simulink subsystem "KinematicModel"  (R2023b)
settings: Solver=VariableStepAuto  StartTime=0.0  StopTime=10.0  RelTol=1e-3
undefined symbols (not defined in the file): EOL_Vehicle_INITR, EOL_Vehicle_InitX, EOL_Vehicle_InitY, EOL_Vehicle_lf, EOL_Vehicle_lr
settings Model: Creator=konur  LastModifiedBy=konur

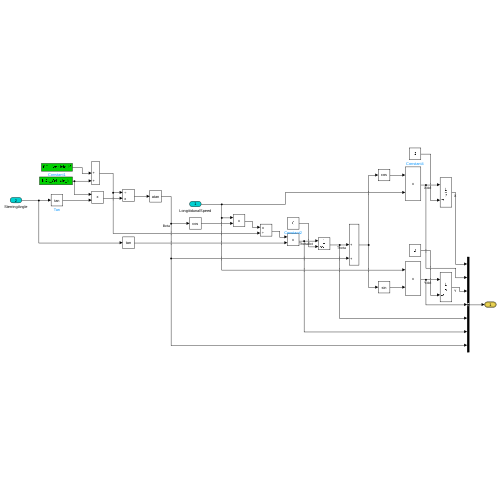
[thumbnail: Simulink's stored preview of the top-level diagram]
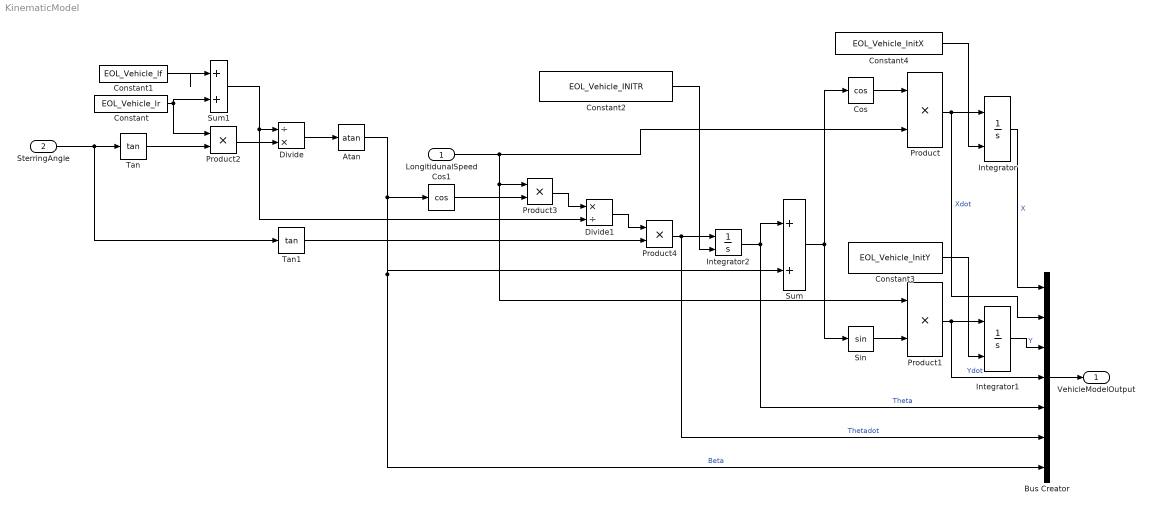
== system KinematicModel ==
  LongitidunalSpeed : Inport
  SterringAngle : Inport  Port=2
  Atan : Trigonometry  Operator=atan
  Bus Creator : BusCreator  Inputs=7  OutDataTypeStr=Bus: VehicleModelBus  NonVirtualBus=on
  Constant : Constant  Value=EOL_Vehicle_lr  OutDataTypeStr=double
  Constant1 : Constant  Value=EOL_Vehicle_lf  OutDataTypeStr=double
  Constant2 : Constant  Value=EOL_Vehicle_INITR  OutDataTypeStr=double
  Constant3 : Constant  Value=EOL_Vehicle_InitY  OutDataTypeStr=double
  Constant4 : Constant  Value=EOL_Vehicle_InitX  OutDataTypeStr=double
  Cos : Trigonometry  Operator=cos
  Cos1 : Trigonometry  Operator=cos
  Divide : Product  Inputs=/*  OutDataTypeStr=double
  Divide1 : Product  Inputs=*/
  Integrator : Integrator  InitialConditionSource=external
  Integrator1 : Integrator  InitialConditionSource=external
  Integrator2 : Integrator  InitialConditionSource=external
  Product{,1..4} (5 alike) : Product
  Sin : Trigonometry
  Sum : Sum  Inputs=|++  OutDataTypeStr=double
  Sum1 : Sum  Inputs=|++  OutDataTypeStr=double
  Tan : Trigonometry  Operator=tan
  Tan1 : Trigonometry  Operator=tan
  VehicleModelOutput : Outport  OutDataTypeStr=Bus: VehicleModelBus
  wires:
  Bus Creator/1 -> VehicleModelOutput/1
  Product1/1 -> Integrator1/1, Bus Creator/4  "Ydot"
  Product/1 -> Integrator/1, Bus Creator/2  "Xdot"
  Constant3/1 -> Integrator1/2
  Cos/1 -> Product/1
  Sum/1 -> Sin/1, Cos/1
  Integrator2/1 -> Sum/1, Bus Creator/5  "Theta"
  Product4/1 -> Integrator2/1, Bus Creator/6  "Thetadot"
  LongitidunalSpeed/1 -> Product3/1, Product1/1, Product/2
  Tan/1 -> Product2/2
  Tan1/1 -> Product4/2
  Constant4/1 -> Integrator/2
  Constant2/1 -> Integrator2/2
  Sum1/1 -> Divide/1, Divide1/2
  Constant/1 -> Sum1/2, Product2/1
  Product2/1 -> Divide/2
  Integrator1/1 -> Bus Creator/3  "Y"
  Sin/1 -> Product1/2
  SterringAngle/1 -> Tan/1, Tan1/1
  Divide/1 -> Atan/1
  Atan/1 -> Sum/2, Bus Creator/7, Cos1/1  "Beta"
  Divide1/1 -> Product4/1
  Constant1/1 -> Sum1/1
  Cos1/1 -> Product3/2
  Integrator/1 -> Bus Creator/1  "X"
  Product3/1 -> Divide1/1
